simulink model "Flight_Simulation"  (R2021b)
settings: Solver=ode4  StartTime=0.0  StopTime=20  FixedStep=Settings.Simulation.step_size  RelTol=1e-3  EnableMultiTasking=on
undefined symbols (not defined in the file or in its folder): AeroCoeff, Aircraft, ControlGains, dLEF, Environment, F, Light, MIL, Settings, Trim, trim_control, trim_state, trim_thrust
libraries: simulink x19, simulink_extras x14, slpidlib x2, aerolibfltsims x2, aerolibwind2 x1, vrlib x1
(part 5 of 5)

== matlab function Flight_Simulation/Non-linear_Plant/Aerodynamic_Modul/Wind to body axis rotation/Wind to body axis rotation ==
  data: Xw input; Yw input; Zw input; Lw input; Mw input; Xb output; Nw input; alfa_rad input; beta_rad input; Yb output; Zb output; Lb output; Mb output; Nb output
function [Xb, Yb, Zb, Lb, Mb, Nb] = fcn(Xw, Yw, Zw, Lw, Mw, Nw, alfa_rad, beta_rad)

% build vectors and matrices
Forces_w = [Xw; Yw; Zw];
Moments_w = [Lw; Mw; Nw];
T_w2b = [cos(alfa_rad)*cos(beta_rad),  -cos(alfa_rad)*sin(beta_rad),  -sin(alfa_rad);...
         sin(beta_rad),                +cos(beta_rad),                 0;...
         sin(alfa_rad)*cos(beta_rad),  -sin(alfa_rad)*sin(beta_rad),  +cos(alfa_rad)];

% transformation
Forces_b = T_w2b * Forces_w;
Moments_b = T_w2b * Moments_w;

% output
Xb = Forces_b(1);
Yb = Forces_b(2);
Zb = Forces_b(3);

Lb = Moments_b(1);
Mb = Moments_b(2);
Nb = Moments_b(3);

end

== matlab function Flight_Simulation/Environment_Subsystems/Wind_Model/Gust_model_(1-cos)/Gust parameters/gust_amplitude_CS-25 ==
  data: H input; h input; U_ds output; Aircraft_Fg input
function U_ds = CS_25_GustAmplitude(H, h, Aircraft_Fg)

% - Based on CS-25 Certification Specification Standard
% - Gust amplitude reference velocity is dependant on the altitude
% - For aeroplane speeds between Vc and Vb

if Aircraft_Fg ~= 0
    F_g     = Aircraft_Fg;   % ---------- flight profile alleviation factor
else
    F_g     = 0.5;
end
H_ref   = 107;   % [m]
h1      = 4572;  % [m]
h2      = 18288; % [m]
U_ref1  = 17.07; % at h=0m [m/s]
U_ref2  = 13.41; % at h=h1 [m/s]
U_ref3  = 6.36;  % at h>h2 [m/s]

if h <= 0 % to make it robust for altitude below sea level
    U_ref = U_ref1;
elseif h < h1
    U_ref = U_ref1 - (U_ref1-U_ref2)./h1 .* h;
elseif h < h2
    U_ref = U_ref2 - (U_ref2-U_ref3)./(h2-h1) .* (h-h1);
else 
    U_ref = U_ref3;
end
    
U_ds = U_ref .* F_g .* (H./H_ref).^(1/6);

end

== matlab function Flight_Simulation/Environment_Subsystems/Wind_Input/wind earth2body trafo ==
  data: Ue input; Uw output; Ve input; We input; phi input; theta input; psi input; Vw output; Ww output
function [Uw,Vw,Ww] = earth2body(Ue, Ve, We, phi, theta, psi)

% pre-caluclations
sphi = sin(phi);
cphi = cos(phi);
spsi = sin(psi);
cpsi = cos(psi);
sthe = sin(theta);
cthe = cos(theta);

% build vectors and matrices
V_earth     = [Ue; Ve; We];
T_e2b       = [cthe*cpsi,                   cthe*spsi,                  -sthe;...
               sphi*sthe*cpsi-cphi*spsi,    sphi*sthe*spsi+cphi*cpsi,   sphi*cthe;...
               cphi*sthe*cpsi+sphi*spsi,    cphi*sthe*spsi-sphi*cpsi,   cphi*cthe];

% calculate
V_body = T_e2b * V_earth;

% output U,V,W
Uw = V_body(1);
Vw = V_body(2);
Ww = V_body(3);

end
